simulink model "cosasdesimulin"  (R2017a)
settings: Solver=VariableStepAuto  StartTime=0.0  StopTime=58  RelTol=1e-3
values from neighbouring files (symbols this model uses):
  denGs = [tau 1]    [control.m]
  numGs = Kest    (= 1.6)    [control.m]
settings Model: Creator=user  LastModifiedBy=user

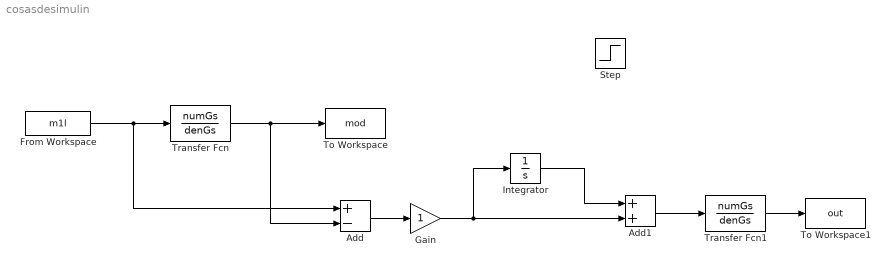
== system cosasdesimulin ==
  Add : Sum  Inputs=+-
  Add1 : Sum
  From Workspace : FromWorkspace  VariableName=m1l
  Gain : Gain
  Integrator : Integrator
  Step : Step  Time=10  Before=136  After=204  SampleTime=0
  To Workspace : ToWorkspace  VariableName=mod  SaveFormat=Timeseries  SampleTime=-1
  To Workspace1 : ToWorkspace  VariableName=out  SaveFormat=Timeseries  SampleTime=-1
  Transfer Fcn : TransferFcn  Numerator=numGs  Denominator=denGs
  Transfer Fcn1 : TransferFcn  Numerator=numGs  Denominator=denGs
  wires:
  Transfer Fcn/1 -> Add/2, To Workspace/1
  From Workspace/1 -> Add/1, Transfer Fcn/1
  Add/1 -> Gain/1
  Gain/1 -> Add1/2, Integrator/1
  Integrator/1 -> Add1/1
  Add1/1 -> Transfer Fcn1/1
  Transfer Fcn1/1 -> To Workspace1/1
